simulink model "Rail_BlkShtCtl"  (R2016b)
settings: configuration reference "CodeGenConfigSet" (kept outside this file)
values from neighbouring files (symbols this model uses):
  Rail_dfrqBlkShtCntDn_C = Calibration.Parameter    [init_Rail_BlkShtCtl.m]    (also in init_Rail_BlkShtCtl_SIL.m = Simulink.Parameter)
  Rail_dfrqBlkShtCntUp_CUR = Calibration.Parameter    [init_Rail_BlkShtCtl.m]    (also in init_Rail_BlkShtCtl_SIL.m = Simulink.Parameter)
  Rail_dfrqBlkShtCntUp_CURX = Calibration.Parameter    [init_Rail_BlkShtCtl.m]    (also in init_Rail_BlkShtCtl_SIL.m = Simulink.Parameter)
  Rail_frqBlkShtDeflate_C = Calibration.Parameter    [init_Rail_BlkShtCtl.m]    (also in init_Rail_BlkShtCtl_SIL.m = Simulink.Parameter)
  Rail_frqBlkShtMax_MAP = Calibration.Parameter    [init_Rail_BlkShtCtl.m]    (also in init_Rail_BlkShtCtl_SIL.m = Simulink.Parameter)
  Rail_frqBlkShtMax_MAPX = Calibration.Parameter    [init_Rail_BlkShtCtl.m]    (also in init_Rail_BlkShtCtl_SIL.m = Simulink.Parameter)
  Rail_frqBlkShtMax_MAPY = Calibration.Parameter    [init_Rail_BlkShtCtl.m]    (also in init_Rail_BlkShtCtl_SIL.m = Simulink.Parameter)
  Rail_frqBlkShtPreCtl_MAP = Calibration.Parameter    [init_Rail_BlkShtCtl.m]    (also in init_Rail_BlkShtCtl_SIL.m = Simulink.Parameter)
  Rail_frqBlkShtPreCtl_MAPX = Calibration.Parameter    [init_Rail_BlkShtCtl.m]    (also in init_Rail_BlkShtCtl_SIL.m = Simulink.Parameter)
  Rail_frqBlkShtPreCtl_MAPY = Calibration.Parameter    [init_Rail_BlkShtCtl.m]    (also in init_Rail_BlkShtCtl_SIL.m = Simulink.Parameter)
  Rail_frqBlkShtThres_C = Calibration.Parameter    [init_Rail_BlkShtCtl.m]    (also in init_Rail_BlkShtCtl_SIL.m = Simulink.Parameter)
  Rail_pBlkShtDeflateHi_C = Calibration.Parameter    [init_Rail_BlkShtCtl.m]    (also in init_Rail_BlkShtCtl_SIL.m = Simulink.Parameter)
  Rail_pBlkShtDeflateLo_C = Calibration.Parameter    [init_Rail_BlkShtCtl.m]    (also in init_Rail_BlkShtCtl_SIL.m = Simulink.Parameter)
  Rail_pBlkShtMax_C = Calibration.Parameter    [init_Rail_BlkShtCtl.m]    (also in init_Rail_BlkShtCtl_SIL.m = Simulink.Parameter)
  Rail_pDvtBlkShtCntDn_C = Calibration.Parameter    [init_Rail_BlkShtCtl.m]    (also in init_Rail_BlkShtCtl_SIL.m = Simulink.Parameter)
  Rail_pDvtBlkShtCntUpHiLim_C = Calibration.Parameter    [init_Rail_BlkShtCtl.m]    (also in init_Rail_BlkShtCtl_SIL.m = Simulink.Parameter)
  Rail_pDvtBlkShtCntUpLoLim_C = Calibration.Parameter    [init_Rail_BlkShtCtl.m]    (also in init_Rail_BlkShtCtl_SIL.m = Simulink.Parameter)
  Rail_qBlkShtStart_C = Calibration.Parameter    [init_Rail_BlkShtCtl.m]    (also in init_Rail_BlkShtCtl_SIL.m = Simulink.Parameter)
  Rail_stCtlBlkShtDeflate_C = Calibration.Parameter    [init_Rail_BlkShtCtl.m]    (also in init_Rail_BlkShtCtl_SIL.m = Simulink.Parameter)
  Rail_stCtlBlkShtOvr_C = Calibration.Parameter    [init_Rail_BlkShtCtl.m]    (also in init_Rail_BlkShtCtl_SIL.m = Simulink.Parameter)
  Rail_swtPh1Byp_C = Calibration.Parameter    [init_Rail_BlkShtCtl.m]    (also in init_Rail_BlkShtCtl_SIL.m = Simulink.Parameter)
  Rail_tiBlkShtCntDn_C = Calibration.Parameter    [init_Rail_BlkShtCtl.m]    (also in init_Rail_BlkShtCtl_SIL.m = Simulink.Parameter)
  Rail_tiBlkShtCntUp_C = Calibration.Parameter    [init_Rail_BlkShtCtl.m]    (also in init_Rail_BlkShtCtl_SIL.m = Simulink.Parameter)
  Rail_tiBlkShtDeflate_C = Calibration.Parameter    [init_Rail_BlkShtCtl.m]    (also in init_Rail_BlkShtCtl_SIL.m = Simulink.Parameter)
undefined symbols (not defined in the file or in its folder): EngState_conv, Rail_BlkShtCtl_DT
libraries: CXLib x3
settings Model: Creator=yangyang  LastModifiedBy=yangyang
settings ConfigSetRef: SourceLocation=Base Workspace

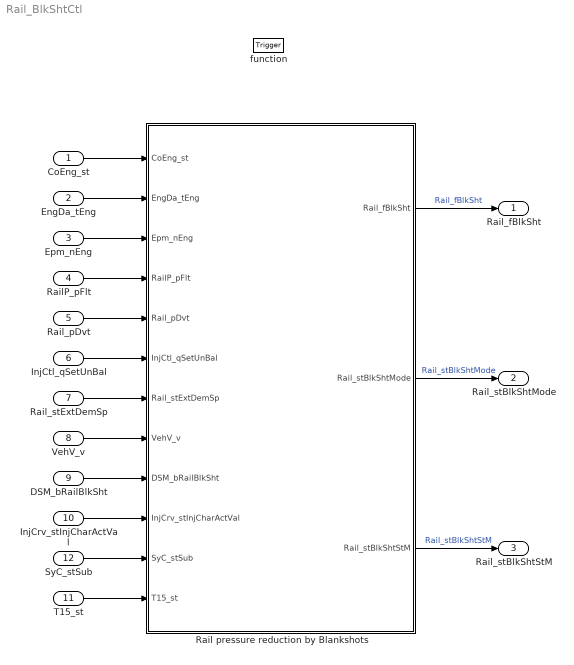
== system Rail_BlkShtCtl ==
  CoEng_st : Inport  Description=Engine operation status  OutDataTypeStr=Enum: EngState_conv
  EngDa_tEng : Inport  Tag=deg  Description=Engine temperature  Port=2  OutMin=-1000  OutMax=1000  OutDataTypeStr=Temp_deg
  Epm_nEng : Inport  Tag=rpm  Description=Engine speed  Port=3  OutMin=0  OutMax=6000  OutDataTypeStr=EngSpeed_rpm
  RailP_pFlt : Inport  Tag=bar  Description=Maximum rail pressure of the last 10 sampling cycle  Port=4  OutMin=0  OutMax=2500  OutDataTypeStr=RailPressure_bar
  Rail_pDvt : Inport  Tag=bar  Description=Governor deviation of the rail pressure governor  Port=5  OutMin=-2500  OutMax=2500  OutDataTypeStr=RailPressure_bar
  InjCtl_qSetUnBal : Inport  Tag=mg/hub  Description=Torque generating engine fuel injection quantity  Port=6  OutMin=-319  OutMax=319  OutDataTypeStr=FuelMass_mg_hub
  Rail_stExtDemSp : Inport  Description=Message to show external interventions on the rail pressure setpoint calculation  Port=7  OutMin=0  OutMax=1  OutDataTypeStr=boolean
  VehV_v : Inport  Tag=km/h  Description=Vehicle speed  Port=8  OutMin=0  OutMax=250  OutDataTypeStr=VehSpeed_km_h
  DSM_bRailBlkSht : Inport  Description=FID for enabling the blank shots in overrun and blank shots for deflating the rail  Port=9  OutMin=0  OutMax=1  OutDataTypeStr=boolean
  InjCrv_stInjCharActVal : Inport  Description=release status of injection types  Port=10  OutMin=0  OutMax=255  OutDataTypeStr=State_uint8
  T15_st : Inport  Description=Terminal 15 status after debouncing  Port=11  OutDataTypeStr=Enum: Switch_conv
  SyC_stSub : Inport  Description=Current system/ECU sub-state  Port=12  OutDataTypeStr=Enum: SubSysExeState_conv
  function : TriggerPort  TriggerType=function-call  VariantControl=Variant
  Rail pressure reduction by Blankshots : Subsystem
  Rail_fBlkSht : Outport  Tag=Hz  Description=Limited blank shot frequency  OutMin=0  OutMax=65535  OutDataTypeStr=Freq_q1p0
  Rail_stBlkShtMode : Outport  Description=Current active blankshot mode  Port=2  OutDataTypeStr=Enum: Rail_BlkShtMode_VERB
  Rail_stBlkShtStM : Outport  Description=State machine for currently active blankshot phase  Port=3  OutDataTypeStr=Enum: Rail_StM_VERB
  wires:
  Rail pressure reduction by Blankshots/1("Rail_fBlkSht ") -> Rail_fBlkSht/1  "Rail_fBlkSht"
  EngDa_tEng/1 -> Rail pressure reduction by Blankshots/2(EngDa_tEng)
  Epm_nEng/1 -> Rail pressure reduction by Blankshots/3(Epm_nEng)
  RailP_pFlt/1 -> Rail pressure reduction by Blankshots/4(RailP_pFlt)
  Rail_pDvt/1 -> Rail pressure reduction by Blankshots/5(Rail_pDvt)
  InjCtl_qSetUnBal/1 -> Rail pressure reduction by Blankshots/6(InjCtl_qSetUnBal)
  Rail_stExtDemSp/1 -> Rail pressure reduction by Blankshots/7(Rail_stExtDemSp)
  VehV_v/1 -> Rail pressure reduction by Blankshots/8(VehV_v)
  DSM_bRailBlkSht/1 -> Rail pressure reduction by Blankshots/9(DSM_bRailBlkSht)
  InjCrv_stInjCharActVal/1 -> Rail pressure reduction by Blankshots/10("InjCrv_stInjCharActVal ")
  CoEng_st/1 -> Rail pressure reduction by Blankshots/1(CoEng_st)
  Rail pressure reduction by Blankshots/2(Rail_stBlkShtMode) -> Rail_stBlkShtMode/1  "Rail_stBlkShtMode"
  Rail pressure reduction by Blankshots/3(Rail_stBlkShtStM) -> Rail_stBlkShtStM/1  "Rail_stBlkShtStM"
  SyC_stSub/1 -> Rail pressure reduction by Blankshots/11(SyC_stSub)
  T15_st/1 -> Rail pressure reduction by Blankshots/12(T15_st)

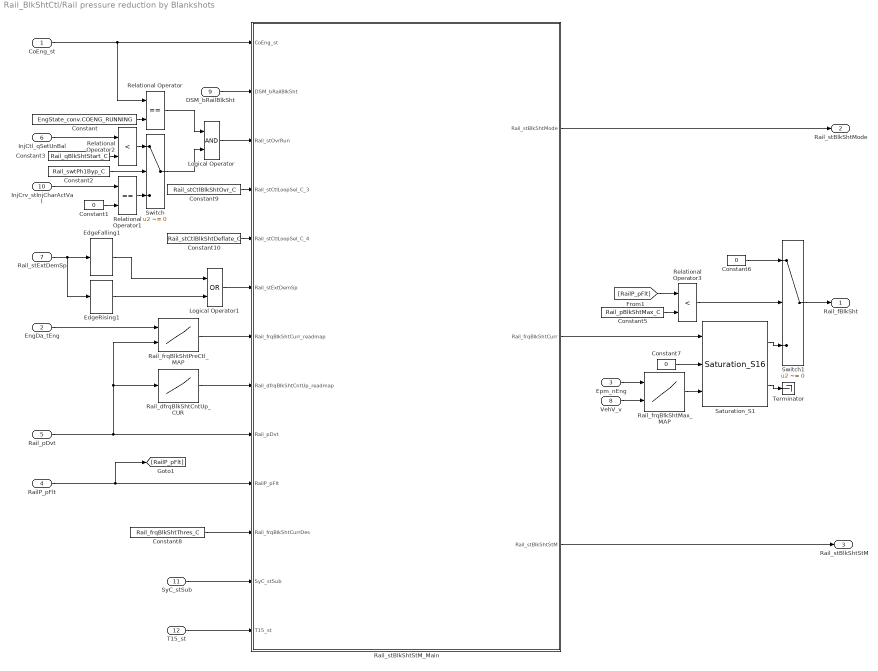
== system Rail_BlkShtCtl/Rail pressure reduction by Blankshots ==
  CoEng_st : Inport
  EngDa_tEng : Inport  Port=2
  Epm_nEng : Inport  Port=3
  RailP_pFlt : Inport  Port=4
  Rail_pDvt : Inport  Port=5
  InjCtl_qSetUnBal : Inport  Port=6
  Rail_stExtDemSp : Inport  Port=7
  VehV_v : Inport  Port=8
  DSM_bRailBlkSht : Inport  Port=9
  "InjCrv_stInjCharActVal " : Inport  Port=10
  SyC_stSub : Inport  Port=11
  T15_st : Inport  Port=12
  Constant : Constant  Value=EngState_conv.COENG_RUNNING  OutDataTypeStr=Inherit: Inherit via back propagation
  Constant1 : Constant  Value=0  OutDataTypeStr=Inherit: Inherit via back propagation
  Constant10 : Constant  Value=Rail_stCtlBlkShtDeflate_C
  Constant2 : Constant  Value=Rail_swtPh1Byp_C
  Constant3 : Constant  Value=Rail_qBlkShtStart_C
  Constant5 : Constant  Value=Rail_pBlkShtMax_C
  Constant6 : Constant  Value=0  OutDataTypeStr=Inherit: Inherit via back propagation
  Constant7 : Constant  Value=0  OutDataTypeStr=Inherit: Inherit via back propagation
  Constant8 : Constant  Value=Rail_frqBlkShtThres_C
  Constant9 : Constant  Value=Rail_stCtlBlkShtOvr_C
  EdgeFalling1 : CXLib/EdgeFalling
  EdgeRising1 : CXLib/EdgeRising
  Logical Operator : Logic  OutDataTypeStr=boolean
  Logical Operator1 : Logic  Operator=OR  OutDataTypeStr=boolean
  Rail_dfrqBlkShtCntUp_CUR : Lookup_n-D  NumberOfTableDimensions=1  BreakpointsForDimension1=Rail_dfrqBlkShtCntUp_CURX  BreakpointsForDimension2=Rail_frqBlkShtPreCtl_MAPX  BreakpointsForDimension3=[5, 7]  BreakpointsForDimension1DataTypeStr=Inherit: Inherit from 'Breakpoint data'  BreakpointsForDimension2DataTypeStr=Inherit: Inherit from 'Breakpoint data'  IndexSearchMethod=Linear search  BeginIndexSearchUsingPreviousIndexResult=on  Table=Rail_dfrqBlkShtCntUp_CUR  TableDataTypeStr=Inherit: Inherit from 'Table data'  ExtrapMethod=Clip  UseLastTableValue=on  InternalRulePriority=Speed  OutDataTypeStr=Inherit: Inherit from 'Table data'  RndMeth=Simplest  SaturateOnIntegerOverflow=on
  Rail_frqBlkShtMax_MAP : Lookup_n-D  BreakpointsForDimension1=Rail_frqBlkShtMax_MAPY  BreakpointsForDimension2=Rail_frqBlkShtMax_MAPX  BreakpointsForDimension3=[5, 7]  BreakpointsForDimension1DataTypeStr=Inherit: Inherit from 'Breakpoint data'  BreakpointsForDimension2DataTypeStr=Inherit: Inherit from 'Breakpoint data'  IndexSearchMethod=Linear search  BeginIndexSearchUsingPreviousIndexResult=on  Table=Rail_frqBlkShtMax_MAP  TableDataTypeStr=Inherit: Inherit from 'Table data'  ExtrapMethod=Clip  UseLastTableValue=on  InternalRulePriority=Speed  OutDataTypeStr=Inherit: Inherit from 'Table data'  RndMeth=Simplest  SaturateOnIntegerOverflow=on
  Rail_frqBlkShtPreCtl_MAP : Lookup_n-D  BreakpointsForDimension1=Rail_frqBlkShtPreCtl_MAPY  BreakpointsForDimension2=Rail_frqBlkShtPreCtl_MAPX  BreakpointsForDimension3=[5, 7]  BreakpointsForDimension1DataTypeStr=Inherit: Inherit from 'Breakpoint data'  BreakpointsForDimension2DataTypeStr=Inherit: Inherit from 'Breakpoint data'  IndexSearchMethod=Linear search  BeginIndexSearchUsingPreviousIndexResult=on  Table=Rail_frqBlkShtPreCtl_MAP  TableDataTypeStr=Inherit: Inherit from 'Table data'  ExtrapMethod=Clip  UseLastTableValue=on  InternalRulePriority=Speed  OutDataTypeStr=Inherit: Inherit from 'Table data'  RndMeth=Simplest  SaturateOnIntegerOverflow=on
  Rail_stBlkShtStM_Main : Stateflow chart  TreatAsAtomicUnit=on
  Relational Operator : RelationalOperator  Operator===  OutDataTypeStr=boolean  RndMeth=Simplest  InputSameDT=on
  Relational Operator1 : RelationalOperator  Operator===  OutDataTypeStr=boolean  RndMeth=Simplest  InputSameDT=on
  Relational Operator2 : RelationalOperator  Operator=<  OutDataTypeStr=boolean  RndMeth=Simplest  InputSameDT=on
  Relational Operator3 : RelationalOperator  Operator=<  OutDataTypeStr=boolean  RndMeth=Simplest  InputSameDT=on
  Saturation_S1 : CXLib/Saturation_S16
  Switch : Switch  Criteria=u2 ~= 0  SaturateOnIntegerOverflow=on  InputSameDT=on
  Switch1 : Switch  Criteria=u2 ~= 0  SaturateOnIntegerOverflow=on  InputSameDT=on
  Terminator : Terminator
  "Rail_fBlkSht " : Outport
  Rail_stBlkShtMode : Outport  Port=2
  Rail_stBlkShtStM : Outport  Port=3
  wires:
  DSM_bRailBlkSht/1 -> Rail_stBlkShtStM_Main/2(DSM_bRailBlkSht)
  CoEng_st/1 -> Rail_stBlkShtStM_Main/1(CoEng_st), Relational Operator/1
  Constant/1 -> Relational Operator/2
  Constant2/1 -> Switch/2
  Relational Operator1/1 -> Switch/3
  Constant1/1 -> Relational Operator1/2
  "InjCrv_stInjCharActVal "/1 -> Relational Operator1/1
  Switch/1 -> Logical Operator/2
  Relational Operator/1 -> Logical Operator/1
  Relational Operator2/1 -> Switch/1
  Constant3/1 -> Relational Operator2/2
  InjCtl_qSetUnBal/1 -> Relational Operator2/1
  Logical Operator/1 -> Rail_stBlkShtStM_Main/3(Rail_stOvrRun)
  Constant9/1 -> Rail_stBlkShtStM_Main/4(Rail_stCtlLoopSel_C_3)
  Constant10/1 -> Rail_stBlkShtStM_Main/5(Rail_stCtlLoopSel_C_4)
  EngDa_tEng/1 -> Rail_frqBlkShtPreCtl_MAP/1
  Rail_pDvt/1 -> Rail_frqBlkShtPreCtl_MAP/2, Rail_dfrqBlkShtCntUp_CUR/1, Rail_stBlkShtStM_Main/9(Rail_pDvt)
  Rail_dfrqBlkShtCntUp_CUR/1 -> Rail_stBlkShtStM_Main/8(Rail_dfrqBlkShtCntUp_readmap)
  Rail_frqBlkShtPreCtl_MAP/1 -> Rail_stBlkShtStM_Main/7(Rail_frqBlkShtCurr_readmap)
  Rail_stExtDemSp/1 -> EdgeRising1/1, EdgeFalling1/1
  EdgeFalling1/1 -> Logical Operator1/1
  EdgeRising1/1 -> Logical Operator1/2
  Logical Operator1/1 -> Rail_stBlkShtStM_Main/6(Rail_stExtDemSp)
  Epm_nEng/1 -> Rail_frqBlkShtMax_MAP/1
  VehV_v/1 -> Rail_frqBlkShtMax_MAP/2
  [RailP_pFlt] -> Relational Operator3/1
  Constant5/1 -> Relational Operator3/2
  Relational Operator3/1 -> Switch1/2
  Switch1/1 -> "Rail_fBlkSht "/1
  Rail_frqBlkShtMax_MAP/1 -> Saturation_S1/3
  Saturation_S1/2 -> Terminator/1
  Constant6/1 -> Switch1/1
  Constant7/1 -> Saturation_S1/2
  Saturation_S1/1 -> Switch1/3
  Rail_stBlkShtStM_Main/2(Rail_frqBlkShtCurr) -> Saturation_S1/1
  Rail_stBlkShtStM_Main/1(Rail_stBlkShtMode) -> Rail_stBlkShtMode/1
  Constant8/1 -> Rail_stBlkShtStM_Main/11(Rail_frqBlkShtCurrDes)
  RailP_pFlt/1 -> [RailP_pFlt], Rail_stBlkShtStM_Main/10(RailP_pFlt)
  Rail_stBlkShtStM_Main/3(Rail_stBlkShtStM) -> Rail_stBlkShtStM/1
  SyC_stSub/1 -> Rail_stBlkShtStM_Main/12(SyC_stSub)
  T15_st/1 -> Rail_stBlkShtStM_Main/13(T15_st)

== stateflow chart Rail_BlkShtCtl/Rail pressure reduction by Blankshots/Rail_stBlkShtStM_Main ==
  state RAIL_STBSPRECTL
    en:Rail_frqBlkShtCurr=Rail_frqBlkShtCurr_readmap;
    Rail_stBlkShtMode=Rail_BlkShtMode_VERB.RAIL_BSOVRRUNDEFLATE;
    Rail_stBlkShtStM=Rail_StM_VERB.RAIL_STBSPRECTL;
    du:Rail_frqBlkShtCurr=Rail_frqBlkShtCurr_readmap;
  state RAIL_STBSREDFREQ
    en:Rail_tiBlkShtCntDn=Rail_BlkShtCtl_DT;
    Rail_stBlkShtStM=Rail_StM_VERB.RAIL_STBSREDFREQ;
    RAIL_STBSREDFREQ -> (junction 28) [order 1]
    (junction 28) -> (junction 25) [order 1] : [Rail_tiBlkShtCntDn<Rail_tiBlkShtCntDn_C*1000]
    (junction 28) -> (junction 31) [order 2] : {Rail_frqBlkShtCurr-=Rail_dfrqBlkShtCntDn_C;
        |  Rail_tiBlkShtCntDn=Rail_BlkShtCtl_DT;}
    (junction 25) -> (junction 27) : {Rail_tiBlkShtCntDn+=Rail_BlkShtCtl_DT;}
    (junction 27) -> (junction 31)
    (junction 31) -> (junction 34)
  state RAIL_STBSINACTV
    en:Rail_frqBlkShtCurr=0;
    Rail_stBlkShtMode=Rail_BlkShtMode_VERB.RAIL_NOBLKSHT;
    Rail_stBlkShtStM=Rail_StM_VERB.RAIL_STBSINACTV;
  state RAIL_STBSDEFLATE
    en:Rail_tiBlkShtDeflate= 0;
    Rail_frqBlkShtCurr=Rail_frqBlkShtDeflate_C;
    Rail_stBlkShtMode=Rail_BlkShtMode_VERB.RAIL_BSAFTRRUN;
    Rail_stBlkShtStM=Rail_StM_VERB.RAIL_STBSDEFLATE;
    du:Rail_frqBlkShtCurr=Rail_frqBlkShtDeflate_C;
    Rail_tiBlkShtDeflate+=Rail_BlkShtCtl_DT;
  state RAIL_STBSSTABILIZE
    en:Rail_tiBlkShtCntUp=Rail_BlkShtCtl_DT;
    Rail_stBlkShtStM=Rail_StM_VERB.RAIL_STBSSTABILIZE;
    du:Rail_dfrqBlkShtCntUp=Rail_dfrqBlkShtCntUp_readmap;
    RAIL_STBSSTABILIZE -> (junction 96) [order 1]
    (junction 96) -> (junction 97) [order 1] : [Rail_pDvt>=Rail_pDvtBlkShtCntUpLoLim_C]
    (junction 96) -> (junction 98) [order 2]
    (junction 97) -> (junction 102)
    (junction 98) -> (junction 99) [order 1] : [Rail_tiBlkShtCntUp<Rail_tiBlkShtCntUp_C*1000]
    (junction 98) -> (junction 100) [order 2] : {Rail_frqBlkShtCurr+=Rail_dfrqBlkShtCntUp;
        |  Rail_tiBlkShtCntUp=Rail_BlkShtCtl_DT;}
    (junction 99) -> (junction 101) : {Rail_tiBlkShtCntUp+=Rail_BlkShtCtl_DT;}
    (junction 101) -> (junction 100)
    (junction 102) -> (junction 101)
    (junction 100) -> (junction 103)
  RAIL_STBSINACTV -> RAIL_STBSPRECTL [order 2] : [Rail_stCtlLoopSel_C_3!=0&&...
      |  Rail_stOvrRun==1&&...
      |  DSM_bRailBlkSht==1&&...
      |  Rail_pDvt<=Rail_pDvtBlkShtCntDn_C]
  RAIL_STBSSTABILIZE -> RAIL_STBSPRECTL [order 1] : [Rail_stOvrRun==1&&...
      |  DSM_bRailBlkSht==1&&...
      |  Rail_pDvt<=Rail_pDvtBlkShtCntUpHiLim_C]
  RAIL_STBSPRECTL -> RAIL_STBSINACTV [order 2] : [Rail_stOvrRun==0||...
      |  DSM_bRailBlkSht==0]
  RAIL_STBSPRECTL -> RAIL_STBSREDFREQ [order 1] : [Rail_stOvrRun==1&&...
      |  DSM_bRailBlkSht==1&&...
      |  Rail_pDvt>Rail_pDvtBlkShtCntDn_C]
  (default) -> RAIL_STBSINACTV
  RAIL_STBSREDFREQ -> RAIL_STBSINACTV [order 2] : [Rail_stOvrRun==0||...
      |  DSM_bRailBlkSht==0||...
      |  Rail_stExtDemSp==1||...
      |  Rail_pDvt>=0]
  RAIL_STBSSTABILIZE -> RAIL_STBSINACTV [order 2] : [Rail_stOvrRun==0||...
      |  DSM_bRailBlkSht==0||...
      |  Rail_stExtDemSp==1||...
      |  Rail_pDvt>=0]
  RAIL_STBSDEFLATE -> RAIL_STBSINACTV : [DSM_bRailBlkSht==0||...
      |  T15_st==Switch_conv.ON||...
      |  SyC_stSub!=SubSysExeState_conv.SYC_POSTDRIVE||...
      |  RailP_pFlt<Rail_pBlkShtDeflateLo_C||...
      |  Rail_tiBlkShtDeflate>Rail_tiBlkShtDeflate_C*1000]
  RAIL_STBSINACTV -> RAIL_STBSDEFLATE [order 1] : [Rail_stCtlLoopSel_C_4!=0&&...
      |  DSM_bRailBlkSht!=0&&...
      |  CoEng_st==EngState_conv.COENG_FINISH&&...
      |  RailP_pFlt>=Rail_pBlkShtDeflateHi_C]
  RAIL_STBSREDFREQ -> RAIL_STBSSTABILIZE [order 1] : [Rail_stOvrRun==1&&...
      |  DSM_bRailBlkSht==1&&...
      |  Rail_frqBlkShtCurr<=Rail_frqBlkShtCurrDes]
  data: CoEng_st input; DSM_bRailBlkSht input; Rail_stOvrRun input; Rail_stCtlLoopSel_C_3 input; Rail_stCtlLoopSel_C_4 input; Rail_stExtDemSp input; Rail_BlkShtCtl_DT parameter; Rail_dfrqBlkShtCntDn_C parameter; Rail_frqBlkShtCurr_readmap input; Rail_dfrqBlkShtCntUp_readmap input; Rail_frqBlkShtDeflate_C parameter; Rail_pDvt input; RailP_pFlt input; Rail_frqBlkShtCurrDes input; Rail_pDvtBlkShtCntDn_C parameter; Rail_pDvtBlkShtCntUpHiLim_C parameter; Rail_pDvtBlkShtCntUpLoLim_C parameter; Rail_tiBlkShtCntDn_C parameter; Rail_tiBlkShtCntUp_C parameter; Rail_tiBlkShtDeflate_C parameter; Rail_stBlkShtMode output Enum: Rail_BlkShtMode_VERB; Rail_dfrqBlkShtCntUp local Freq_q1p0; Rail_frqBlkShtCurr output; Rail_tiBlkShtCntDn local Debounce_ms; Rail_tiBlkShtCntUp local Debounce_ms; Rail_tiBlkShtDeflate local Debounce_ms; Rail_pBlkShtDeflateHi_C parameter; Rail_pBlkShtDeflateLo_C parameter double; SyC_stSub input; T15_st input; Rail_stBlkShtStM output Enum: Rail_StM_VERB
